simulink model "Duggoff_Tire_Model"  (R2022b)
settings: Solver=VariableStepAuto  StartTime=0.0  StopTime=100  RelTol=1e-3
undefined symbols (not defined in the file): alpha, C_x, C_y, Fzf, mu, s
settings Model: Creator=Samsung  LastModifiedBy=brianlesko
settings SolverCC: AlgebraicLoopSolver=TrustRegion
settings DataIOCC: ReturnWorkspaceOutputs=off
settings DebuggingCC: UnconnectedInputMsg=warning  UnconnectedOutputMsg=warning  UnconnectedLineMsg=warning  SFMachineParentedDataDiag=warning  ArithmeticOperatorsInVariantConditions=warning
settings ModelReferenceCC: EnableRefExpFcnMdlSchedulingChecks=on
settings SFSimCC: SimUseLocalCustomCode=off  CustomCodeUndefinedFunction=UseInterfaceOnly
settings RTWCC: RTWUseLocalCustomCode=off
settings CodeAppCC: StateflowObjectComments=on
settings SimscapeCC: SimscapeNormalizeSystem=off

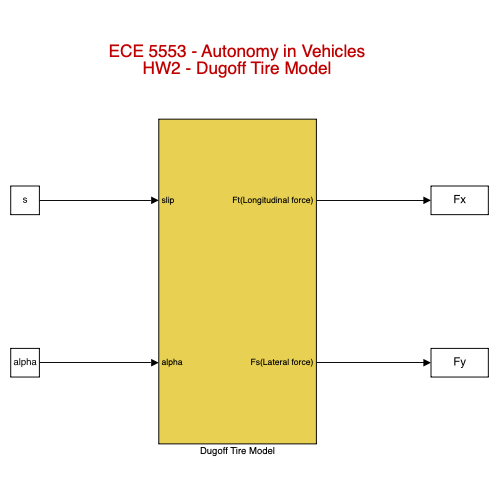
[thumbnail: Simulink's stored preview of the top-level diagram]
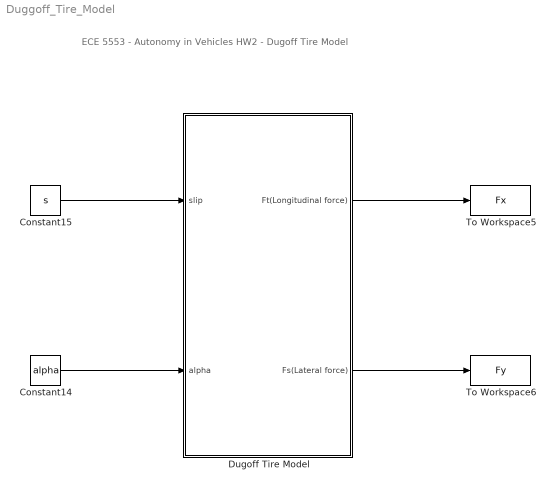
== system Duggoff_Tire_Model ==
  note: ECE 5553 - Autonomy in Vehicles
      | HW2 - Dugoff Tire Model
  Constant14 : Constant  Value=alpha  OutDataTypeStr=single
  Constant15 : Constant  Value=s
  Dugoff Tire Model : Subsystem
  To Workspace5 : ToWorkspace  VariableName=Fx  SampleTime=-1
  To Workspace6 : ToWorkspace  VariableName=Fy  SampleTime=-1
  wires:
  Constant15/1 -> Dugoff Tire Model/1(slip)
  Dugoff Tire Model/1(Ft(Longitudinal force)) -> To Workspace5/1
  Constant14/1 -> Dugoff Tire Model/2(alpha)
  Dugoff Tire Model/2(Fs(Lateral force)) -> To Workspace6/1

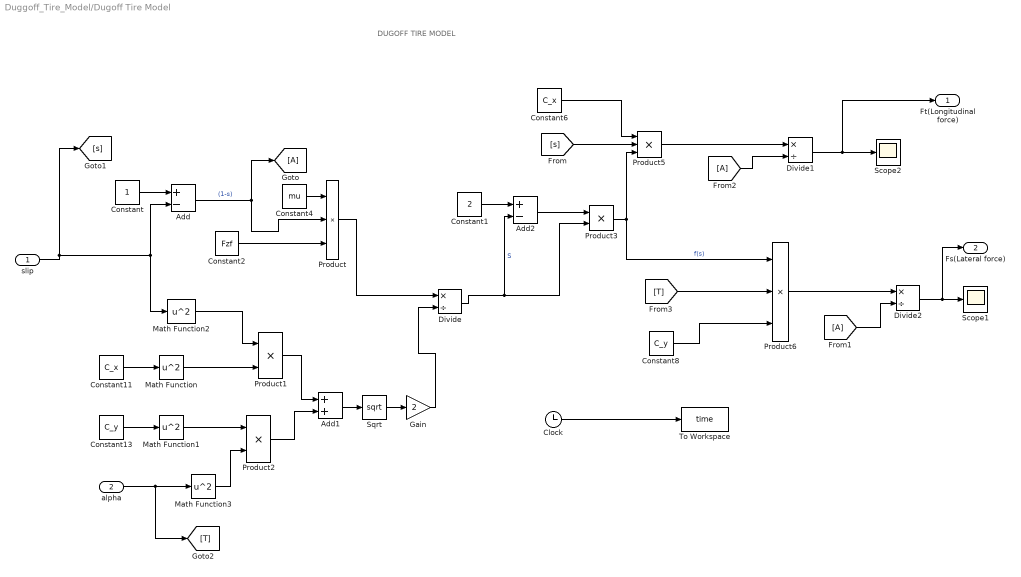
== system Duggoff_Tire_Model/Dugoff Tire Model ==
  note: DUGOFF TIRE MODEL
  slip : Inport
  alpha : Inport  Port=2
  Add : Sum  Inputs=+-
  Add1 : Sum
  Add2 : Sum  Inputs=+-
  Clock : Clock
  Constant : Constant
  Constant1 : Constant  Value=2
  Constant11 : Constant  Value=C_x
  Constant13 : Constant  Value=C_y
  Constant2 : Constant  Value=Fzf
  Constant4 : Constant  Value=mu
  Constant6 : Constant  Value=C_x
  Constant8 : Constant  Value=C_y
  Divide : Product  Inputs=*/
  Divide1 : Product  Inputs=*/
  Divide2 : Product  Inputs=*/
  From1 : From
  From2 : From
  Gain : Gain  Gain=2
  Goto : Goto
  Math Function{,1..3} (4 alike) : Math  Operator=square  SignedPower=on
  Product : Product  Inputs=3
  Product1 : Product
  Product2 : Product
  Product3 : Product
  Product5 : Product  Inputs=3
  Product6 : Product  Inputs=3
  Scope1 : Scope
  Scope2 : Scope
  Sqrt : Sqrt
  To Workspace : ToWorkspace  VariableName=time  SampleTime=-1
  Ft(Longitudinal force) : Outport  VectorParamsAs1DForOutWhenUnconnected=off
  Fs(Lateral force) : Outport  Port=2  VectorParamsAs1DForOutWhenUnconnected=off
  wires:
  Constant11/1 -> Math Function/1
  Math Function3/1 -> Product2/2
  Sqrt/1 -> Gain/1
  From1/1 -> Divide2/2
  Math Function1/1 -> Product2/1
  alpha/1 -> [T], Math Function3/1
  Gain/1 -> Divide/2
  Constant8/1 -> Product6/3
  Clock/1 -> To Workspace/1
  Constant1/1 -> Add2/1
  From2/1 -> Divide1/2
  [T] -> Product6/2
  [s] -> Product5/2
  Math Function/1 -> Product1/2
  slip/1 -> [s], Math Function2/1, Add/2
  Constant2/1 -> Product/3
  Add/1 -> Product/2, Goto/1  "(1-s)"
  Product5/1 -> Divide1/1
  Divide/1 -> Product3/2, Add2/2  "S"
  Product3/1 -> Product6/1, Product5/3  "f(s)"
  Add2/1 -> Product3/1
  Divide2/1 -> Fs(Lateral force)/1, Scope1/1
  Divide1/1 -> Ft(Longitudinal force)/1, Scope2/1
  Product1/1 -> Add1/1
  Constant/1 -> Add/1
  Constant4/1 -> Product/1
  Add1/1 -> Sqrt/1
  Constant13/1 -> Math Function1/1
  Math Function2/1 -> Product1/1
  Product6/1 -> Divide2/1
  Product/1 -> Divide/1
  Constant6/1 -> Product5/1
  Product2/1 -> Add1/2
